simulink model "PowerFlow_SUSAN"  (R2021b)
settings: Solver=FixedStepAuto  StartTime=0.0  StopTime=10  FixedStep=0.02  RelTol=1e-3
undefined symbols (not defined in the file): MWS
libraries: Lib_EMTAT x193
(part 3 of 3)

== system PowerFlow_SUSAN/Bus System 4/Propulsor System 3 ==
  Iin : Inport
  Tset : Inport  Port=2
  Bus Selector : BusSelector  OutputSignals=T
  Bus Selector1 : BusSelector  OutputSignals=Tset 4-3-1,Tset 4-3-2
  Bus Selector2 : BusSelector  OutputSignals=T
  Cable1 : Lib_EMTAT/Components/Power Flow/Cable  R_c=0.2
      settings: SourceProductName=EMTAT
  Cable3 : Lib_EMTAT/Components/Power Flow/Cable  R_c=0.2
      settings: SourceProductName=EMTAT
  Constant2 : Constant  Value=350
  Current Junction : Lib_EMTAT/Components/Power Flow/Current Junction
      settings: SourceProductName=EMTAT
      settings: AttributesFormatString=|
      | Current Junction
      | Version: %<LibraryVersion>
  DC-DC Converter : Lib_EMTAT/Components/Power Flow/DC-DC Converter  X_Vout_VoltageVec_M=[0 100 1000 5000]  Y_Iout_CurrentVec_M=[0 10 100 150]  T_C_EffArray_M=0.98*ones(4,4)
      settings: SourceProductName=EMTAT
  Display9 : Display
  Integrator1 : Integrator  InitialCondition=150
  Integrator2 : Integrator  InitialCondition=2000
  Integrator3 : Integrator  InitialCondition=2000
  Inverter/Rectifier (Sink)1 : Lib_EMTAT/Components/Power Flow/Inverter//Rectifier (Sink)  X_C_VoltageInVec_M=MWS.I1.Vdc  Y_C_RMSCurrentOutVec_M=MWS.I1.Irms  T_C_PowLossArray_M=MWS.I1.Ploss'  K_e=0.0503
      settings: SourceProductName=EMTAT
  Inverter/Rectifier (Sink)2 : Lib_EMTAT/Components/Power Flow/Inverter//Rectifier (Sink)  X_C_VoltageInVec_M=MWS.I1.Vdc  Y_C_RMSCurrentOutVec_M=MWS.I1.Irms  T_C_PowLossArray_M=MWS.I1.Ploss'  K_e=0.0503
      settings: SourceProductName=EMTAT
  Mechanical Shaft1 : Lib_EMTAT/Components/Power Flow/Mechanical Shaft  J=0.01  B=0.001
      settings: SourceProductName=EMTAT
  Mechanical Shaft2 : Lib_EMTAT/Components/Power Flow/Mechanical Shaft  J=0.01  B=0.001
      settings: SourceProductName=EMTAT
  Motor/Generator (Sink)1 : Lib_EMTAT/Components/Power Flow/Motor//Generator (Sink)  X_C_SpeedVec_M=[0 100 1000 5000]  Y_C_TorqueVec_M=[0 10 100 150]  T_C_EffArray_M=0.99*ones(4,4)
      settings: SourceProductName=EMTAT
  Motor/Generator (Sink)3 : Lib_EMTAT/Components/Power Flow/Motor//Generator (Sink)  X_C_SpeedVec_M=[0 100 1000 5000]  Y_C_TorqueVec_M=[0 10 100 150]  T_C_EffArray_M=0.99*ones(4,4)
      settings: SourceProductName=EMTAT
  Mux : Mux  Inputs=2
  Mux1 : Mux  Inputs=2
  Sum of Elements : Sum  Inputs=+
  Super Capacitor : Lib_EMTAT/Components/Power Flow/Energy Storage Device  C=130  ESR=0.02  TSE=0
      settings: SourceProductName=EMTAT
  Terminator{1..6,8,11..13,17..24} (18 alike) : Terminator
  Unit Delay1 : UnitDelay  SampleTime=-1  HasFrameUpgradeWarning=on
  Unit Delay2 : UnitDelay  SampleTime=-1  HasFrameUpgradeWarning=on
  Unit Delay3 : UnitDelay  SampleTime=-1  HasFrameUpgradeWarning=on
  Vout : Outport
  Idmd : Outport  Port=2
  wires:
  Tset/1 -> Bus Selector1/1
  Bus Selector1/2 -> [Tset_2]  "<Tset 4-3-2>"
  Bus Selector1/1 -> [Tset_1]  "<Tset 4-3-1>"
  Sum of Elements/1 -> Idmd/1, Mux/2
  Mux1/1 -> Sum of Elements/1
  Bus Selector/1 -> Mechanical Shaft1/1  "<T>"
  Inverter/Rectifier (Sink)1/2 -> Terminator5/1
  Motor/Generator (Sink)3/1 -> Bus Selector2/1
  [Tset_2] -> Motor/Generator (Sink)3/3
  DC-DC Converter/3 -> Terminator23/1
  DC-DC Converter/2 -> Terminator22/1
  Mechanical Shaft1/2 -> Terminator17/1
  [N_M2] -> Inverter/Rectifier (Sink)2/2
  Inverter/Rectifier (Sink)2/4 -> Cable3/2
  Motor/Generator (Sink)3/2 -> Terminator21/1
  Super Capacitor/3 -> Terminator12/1
  Cable1/2 -> Terminator18/1
  Bus Selector2/1 -> Mechanical Shaft2/1  "<T>"
  Cable3/3 -> Terminator3/1
  Motor/Generator (Sink)1/2 -> Terminator8/1
  Constant2/1 -> DC-DC Converter/1
  Cable1/4 -> Mux1/1
  Unit Delay1/1 -> Super Capacitor/3
  Super Capacitor/5 -> Unit Delay1/1
  Inverter/Rectifier (Sink)1/3 -> Terminator6/1
  Cable1/5 -> Unit Delay2/1
  Mechanical Shaft2/2 -> Terminator1/1
  Integrator1/1 -> Super Capacitor/2
  Inverter/Rectifier (Sink)1/4 -> Cable1/2
  Unit Delay3/1 -> Cable3/3
  Motor/Generator (Sink)3/3 -> Inverter/Rectifier (Sink)2/3
  Cable1/3 -> Terminator19/1
  Inverter/Rectifier (Sink)2/2 -> Terminator20/1
  Inverter/Rectifier (Sink)2/1 -> Motor/Generator (Sink)3/1
  Integrator3/1 -> [N_M2], Mechanical Shaft2/2
  Cable3/4 -> Mux1/2
  Super Capacitor/2 -> Terminator11/1
  Inverter/Rectifier (Sink)2/3 -> Terminator4/1
  Mechanical Shaft2/3 -> Terminator24/1
  Inverter/Rectifier (Sink)1/1 -> Display9/1, Motor/Generator (Sink)1/1
  Cable3/5 -> Unit Delay3/1
  [N_M1] -> Inverter/Rectifier (Sink)1/2
  Cable1/1 -> Inverter/Rectifier (Sink)1/1
  Motor/Generator (Sink)1/1 -> Bus Selector/1
  Integrator2/1 -> [N_M1], Mechanical Shaft1/2
  Mux/1 -> Current Junction/1
  Current Junction/1 -> DC-DC Converter/3
  DC-DC Converter/4 -> Super Capacitor/1
  Cable3/2 -> Terminator2/1
  Unit Delay2/1 -> Cable1/3
  Mechanical Shaft1/3 -> Terminator13/1
  [N_M1] -> Motor/Generator (Sink)1/2
  Cable3/1 -> Inverter/Rectifier (Sink)2/1
  Super Capacitor/1 -> DC-DC Converter/2
  Super Capacitor/4 -> Integrator1/1
  Motor/Generator (Sink)1/3 -> Inverter/Rectifier (Sink)1/3
  Mechanical Shaft1/1 -> Integrator2/1
  DC-DC Converter/1 -> Cable1/1, Vout/1, Cable3/1
  [N_M2] -> Motor/Generator (Sink)3/2
  [Tset_1] -> Motor/Generator (Sink)1/3
  Mechanical Shaft2/1 -> Integrator3/1
  Iin/1 -> Mux/1

== system PowerFlow_SUSAN/Bus System 4/Propulsor System 4 ==
  Iin : Inport
  Tset : Inport  Port=2
  Bus Selector : BusSelector  OutputSignals=T
  Bus Selector1 : BusSelector  OutputSignals=Tset 4-4-1,Tset 4-4-2
  Bus Selector2 : BusSelector  OutputSignals=T
  Cable1 : Lib_EMTAT/Components/Power Flow/Cable  R_c=0.2
      settings: SourceProductName=EMTAT
  Cable3 : Lib_EMTAT/Components/Power Flow/Cable  R_c=0.2
      settings: SourceProductName=EMTAT
  Constant2 : Constant  Value=350
  Current Junction : Lib_EMTAT/Components/Power Flow/Current Junction
      settings: SourceProductName=EMTAT
      settings: AttributesFormatString=|
      | Current Junction
      | Version: %<LibraryVersion>
  DC-DC Converter : Lib_EMTAT/Components/Power Flow/DC-DC Converter  X_Vout_VoltageVec_M=[0 100 1000 5000]  Y_Iout_CurrentVec_M=[0 10 100 150]  T_C_EffArray_M=0.98*ones(4,4)
      settings: SourceProductName=EMTAT
  Display9 : Display
  Integrator1 : Integrator  InitialCondition=150
  Integrator2 : Integrator  InitialCondition=2000
  Integrator3 : Integrator  InitialCondition=2000
  Inverter/Rectifier (Sink)1 : Lib_EMTAT/Components/Power Flow/Inverter//Rectifier (Sink)  X_C_VoltageInVec_M=MWS.I1.Vdc  Y_C_RMSCurrentOutVec_M=MWS.I1.Irms  T_C_PowLossArray_M=MWS.I1.Ploss'  K_e=0.0503
      settings: SourceProductName=EMTAT
  Inverter/Rectifier (Sink)2 : Lib_EMTAT/Components/Power Flow/Inverter//Rectifier (Sink)  X_C_VoltageInVec_M=MWS.I1.Vdc  Y_C_RMSCurrentOutVec_M=MWS.I1.Irms  T_C_PowLossArray_M=MWS.I1.Ploss'  K_e=0.0503
      settings: SourceProductName=EMTAT
  Mechanical Shaft1 : Lib_EMTAT/Components/Power Flow/Mechanical Shaft  J=0.01  B=0.001
      settings: SourceProductName=EMTAT
  Mechanical Shaft2 : Lib_EMTAT/Components/Power Flow/Mechanical Shaft  J=0.01  B=0.001
      settings: SourceProductName=EMTAT
  Motor/Generator (Sink)1 : Lib_EMTAT/Components/Power Flow/Motor//Generator (Sink)  X_C_SpeedVec_M=[0 100 1000 5000]  Y_C_TorqueVec_M=[0 10 100 150]  T_C_EffArray_M=0.99*ones(4,4)
      settings: SourceProductName=EMTAT
  Motor/Generator (Sink)3 : Lib_EMTAT/Components/Power Flow/Motor//Generator (Sink)  X_C_SpeedVec_M=[0 100 1000 5000]  Y_C_TorqueVec_M=[0 10 100 150]  T_C_EffArray_M=0.99*ones(4,4)
      settings: SourceProductName=EMTAT
  Mux : Mux  Inputs=2
  Mux1 : Mux  Inputs=2
  Sum of Elements : Sum  Inputs=+
  Super Capacitor : Lib_EMTAT/Components/Power Flow/Energy Storage Device  C=130  ESR=0.02  TSE=0
      settings: SourceProductName=EMTAT
  Terminator{1..6,8,11..13,17..24} (18 alike) : Terminator
  Unit Delay1 : UnitDelay  SampleTime=-1  HasFrameUpgradeWarning=on
  Unit Delay2 : UnitDelay  SampleTime=-1  HasFrameUpgradeWarning=on
  Unit Delay3 : UnitDelay  SampleTime=-1  HasFrameUpgradeWarning=on
  Vout : Outport
  Idmd : Outport  Port=2
  wires:
  Iin/1 -> Mux/1
  Mechanical Shaft2/1 -> Integrator3/1
  [Tset_1] -> Motor/Generator (Sink)1/3
  [N_M2] -> Motor/Generator (Sink)3/2
  DC-DC Converter/1 -> Cable3/1, Vout/1, Cable1/1
  Mechanical Shaft1/1 -> Integrator2/1
  Motor/Generator (Sink)1/3 -> Inverter/Rectifier (Sink)1/3
  Super Capacitor/4 -> Integrator1/1
  Super Capacitor/1 -> DC-DC Converter/2
  Cable3/1 -> Inverter/Rectifier (Sink)2/1
  [N_M1] -> Motor/Generator (Sink)1/2
  Mechanical Shaft1/3 -> Terminator13/1
  Unit Delay2/1 -> Cable1/3
  Cable3/2 -> Terminator2/1
  DC-DC Converter/4 -> Super Capacitor/1
  Current Junction/1 -> DC-DC Converter/3
  Mux/1 -> Current Junction/1
  Integrator2/1 -> Mechanical Shaft1/2, [N_M1]
  Motor/Generator (Sink)1/1 -> Bus Selector/1
  Cable1/1 -> Inverter/Rectifier (Sink)1/1
  [N_M1] -> Inverter/Rectifier (Sink)1/2
  Cable3/5 -> Unit Delay3/1
  Inverter/Rectifier (Sink)1/1 -> Motor/Generator (Sink)1/1, Display9/1
  Mechanical Shaft2/3 -> Terminator24/1
  Inverter/Rectifier (Sink)2/3 -> Terminator4/1
  Super Capacitor/2 -> Terminator11/1
  Cable3/4 -> Mux1/2
  Integrator3/1 -> Mechanical Shaft2/2, [N_M2]
  Inverter/Rectifier (Sink)2/1 -> Motor/Generator (Sink)3/1
  Inverter/Rectifier (Sink)2/2 -> Terminator20/1
  Cable1/3 -> Terminator19/1
  Motor/Generator (Sink)3/3 -> Inverter/Rectifier (Sink)2/3
  Unit Delay3/1 -> Cable3/3
  Inverter/Rectifier (Sink)1/4 -> Cable1/2
  Integrator1/1 -> Super Capacitor/2
  Mechanical Shaft2/2 -> Terminator1/1
  Cable1/5 -> Unit Delay2/1
  Inverter/Rectifier (Sink)1/3 -> Terminator6/1
  Super Capacitor/5 -> Unit Delay1/1
  Unit Delay1/1 -> Super Capacitor/3
  Cable1/4 -> Mux1/1
  Constant2/1 -> DC-DC Converter/1
  Motor/Generator (Sink)1/2 -> Terminator8/1
  Cable3/3 -> Terminator3/1
  Bus Selector2/1 -> Mechanical Shaft2/1  "<T>"
  Cable1/2 -> Terminator18/1
  Super Capacitor/3 -> Terminator12/1
  Motor/Generator (Sink)3/2 -> Terminator21/1
  Inverter/Rectifier (Sink)2/4 -> Cable3/2
  [N_M2] -> Inverter/Rectifier (Sink)2/2
  Mechanical Shaft1/2 -> Terminator17/1
  DC-DC Converter/2 -> Terminator22/1
  DC-DC Converter/3 -> Terminator23/1
  [Tset_2] -> Motor/Generator (Sink)3/3
  Motor/Generator (Sink)3/1 -> Bus Selector2/1
  Inverter/Rectifier (Sink)1/2 -> Terminator5/1
  Bus Selector/1 -> Mechanical Shaft1/1  "<T>"
  Mux1/1 -> Sum of Elements/1
  Sum of Elements/1 -> Mux/2, Idmd/1
  Bus Selector1/1 -> [Tset_1]  "<Tset 4-4-1>"
  Bus Selector1/2 -> [Tset_2]  "<Tset 4-4-2>"
  Tset/1 -> Bus Selector1/1
